simulink model "DSB-SC Modulation and Demodulation"  (R2021a)
settings: Solver=VariableStepAuto  StartTime=0.0  StopTime=2  RelTol=1e-3
libraries: dspsrcs4 x2, eeGeneralControl x1
settings Model: Creator=mluser  LastModifiedBy=mluser
settings SolverCC: AlgebraicLoopSolver=TrustRegion
settings DebuggingCC: SFMachineParentedDataDiag=warning

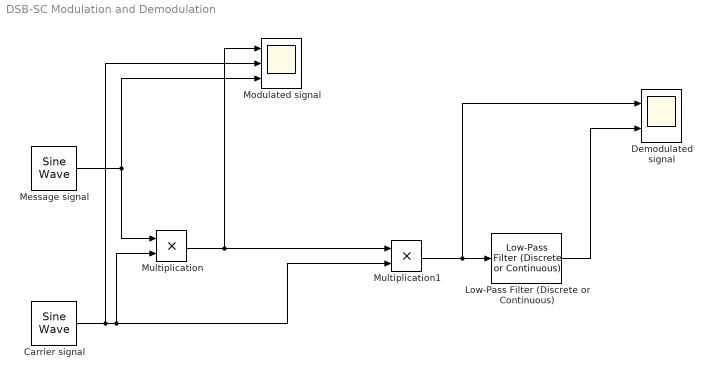
== system DSB-SC Modulation and Demodulation ==
  Carrier signal : dspsrcs4/Sine Wave  Amplitude=1  Frequency=20  Phase=0  SampleMode=Continuous  OutComplex=Real  CompMethod=Trigonometric fcn  TableSize=Speed  SampleTime=1/1000  SamplesPerFrame=1  ResetState=Restart at time zero  OutputFrames=off  dataType=double  wordLen=16  udDataType=sfix(16)  fracBitsMode=Best precision  numFracBits=15  OutDataTypeStr=double  LastOutDataTypeStr=double
  Demodulated signal : Scope  NumInputPorts=2
  Low-Pass Filter (Discrete or Continuous) : eeGeneralControl/Low-Pass Filter (Discrete or Continuous)  K=16/6  T=1/6  B=inf  A=-inf  init_option=Specify as parameter  x0=0  Ts=1/1000
  Message signal : dspsrcs4/Sine Wave  Amplitude=1  Frequency=1  Phase=0  SampleMode=Continuous  OutComplex=Real  CompMethod=Trigonometric fcn  TableSize=Speed  SampleTime=1/1000  SamplesPerFrame=1  ResetState=Restart at time zero  OutputFrames=off  dataType=double  wordLen=16  udDataType=sfix(16)  fracBitsMode=Best precision  numFracBits=15  OutDataTypeStr=double  LastOutDataTypeStr=double
  Modulated signal : Scope  NumInputPorts=3
  Multiplication : Product
  Multiplication1 : Product
  wires:
  Carrier signal/1 -> Modulated signal/2, Multiplication1/2, Multiplication/2
  Message signal/1 -> Multiplication/1, Modulated signal/3
  Multiplication/1 -> Multiplication1/1, Modulated signal/1
  Multiplication1/1 -> Low-Pass Filter (Discrete or Continuous)/1, Demodulated signal/1
  Low-Pass Filter (Discrete or Continuous)/1 -> Demodulated signal/2
